simulink model "SHEST"  (R2022a)
settings: Solver=ode23tb  StartTime=0.0  StopTime=0.1  MaxStep=1e-3  RelTol=1e-2
undefined symbols (not defined in the file): DC_Source, Modulation_Index, phase_3_IGBTs, Sine_Wave, Three_Phase_RL
libraries: spsFourierLib x4, spsVoltageMeasurementLib x3, spsCurrentMeasurementLib x2, spsUniversalBridgeLib x1, spsDCVoltageSourceLib x1, spsMultimeterLib x1, spsPWMGenerator2LevelLib x1, spsRMSLib x1, spsThreePhaseSeriesRLCBranchLib x1, spspowerguiLib x1
settings Model: Creator=Student11  LastModifiedBy=админ
settings SolverCC: AlgebraicLoopSolver=TrustRegion
settings DataIOCC: ReturnWorkspaceOutputs=off
settings DebuggingCC: SFMachineParentedDataDiag=warning  ArithmeticOperatorsInVariantConditions=warning
settings SFSimCC: SimUseLocalCustomCode=off  CustomCodeUndefinedFunction=UseInterfaceOnly
settings RTWCC: RTWUseLocalCustomCode=off
settings CodeAppCC: StateflowObjectComments=on
settings SimscapeCC: SimscapeNormalizeSystem=off

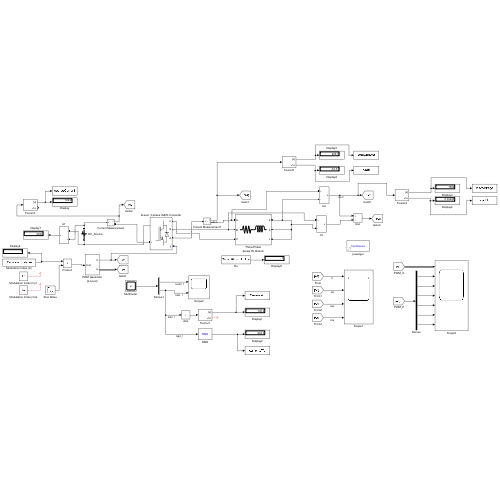
[thumbnail: Simulink's stored preview of the top-level diagram]
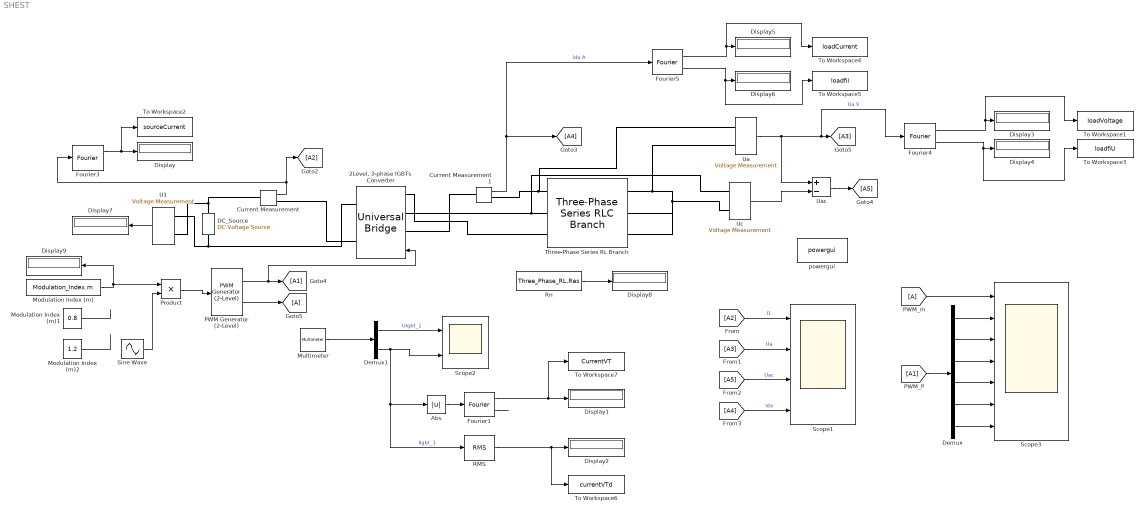
== system SHEST ==
  "2Level, 3-phase IGBTs Converter" : spsUniversalBridgeLib/Universal Bridge  Arms=3  SnubberResistance=phase_3_IGBTs.SnubberRs  SnubberCapacitance=phase_3_IGBTs.SnubberCs  Device=IGBT / Diodes  Ron=phase_3_IGBTs.R_on  Lon=0  ForwardVoltages=[phase_3_IGBTs.Vf phase_3_IGBTs.Vfd]  ForwardVoltage=[2 1]  GTOparameters=[ 10e-6 , 20e-6 ]  IGBTparameters=[ 1e-6 , 2e-6 ]  Measurements=All voltages and currents  Measurements_2=None  converterType=Rectifier
  Abs : Abs  SaturateOnIntegerOverflow=off
  Current Measurement : spsCurrentMeasurementLib/Current Measurement  PhasorSimulation=off  OutputType=Complex  PSBequivalent=0
  Current Measurement1 : spsCurrentMeasurementLib/Current Measurement  PhasorSimulation=off  OutputType=Complex  PSBequivalent=0
  DC_Source : spsDCVoltageSourceLib/DC Voltage Source  Amplitude=DC_Source.Voltage  Measurements=None
  Demux : Demux  Outputs=6
  Demux1 : Demux  Outputs=2
  Display{,1..9} (10 alike) : Display
  Fourier1 : spsFourierLib/Fourier  Freq=Fourier_1_4_5.frec  n=Fourier_1_4_5.harmonic  InInit=[0, 0]  Ts=0
      settings: SourceProductBaseCode=PS
  Fourier3 : spsFourierLib/Fourier  Freq=Fourier_3.frec  n=Fourier_3.harmonic  InInit=[0, 0]  Ts=0
      settings: SourceProductBaseCode=PS
  Fourier4 : spsFourierLib/Fourier  Freq=Fourier_1_4_5.frec  n=Fourier_1_4_5.harmonic  InInit=[0, 0]  Ts=0
      settings: SourceProductBaseCode=PS
  Fourier5 : spsFourierLib/Fourier  Freq=Fourier_1_4_5.frec  n=Fourier_1_4_5.harmonic  InInit=[0, 0]  Ts=0
      settings: SourceProductBaseCode=PS
  Goto5 : Goto
  Modulation Index (m) : Constant  Value=Modulation_Index.m
  Modulation Index (m)1 : Constant  Value=0.8
  Modulation Index (m)2 : Constant  Value=1.2
  Multimeter : spsMultimeterLib/Multimeter  L=16  sel=[1 11]  yselected={}  Gain=[1 1]  OutputType=Complex  PlotAtSimulationStop=off  PhasorSimulation=off
  PWM Generator (2-Level) : spsPWMGenerator2LevelLib/PWM Generator (2-Level)  ModulatorType=Three-phase bridge (6 pulses)  ModulatorMode=Unsynchronized  Fc=PWM_generator.frec  Pc=0  nF=27  MinMax="[ -1  1 ]"  SamplingTechnique=Natural  ModulatingSignals=off  m=0.8  Freq=60  Phase=0  Ts=0  ShowCarrierOutport=on
  PWM_m : From
  Product : Product
  RMS : spsRMSLib/RMS  TrueRMS=on  Freq=RMS_T.frec  RMSInit=0  Ts=0
  Rн : Constant  Value=Three_Phase_RL.Res
  Scope1 : Scope  NumInputPorts=4
  Scope2 : Scope  NumInputPorts=2
  Scope3 : Scope  NumInputPorts=7
  Sine Wave : Sin  Amplitude=Sine_Wave.amplitude  Frequency=Sine_Wave.freq  Phase=Sine_Wave.Phase  SampleTime=0
  Three-Phase Series RL Branch : spsThreePhaseSeriesRLCBranchLib/Three-Phase Series RLC Branch  LConnTagsString=A|B|C  RConnTagsString=A|B|C  BranchType=RL  Resistance=Three_Phase_RL.Res  Inductance=Three_Phase_RL.Ind  Capacitance=1e-6  Measurements=None
  To Workspace1 : ToWorkspace  VariableName=loadVoltage  SampleTime=-1
  To Workspace2 : ToWorkspace  VariableName=sourceCurrent  SampleTime=-1
  To Workspace3 : ToWorkspace  VariableName=loadfiU  SampleTime=-1
  To Workspace4 : ToWorkspace  VariableName=loadCurrent  SampleTime=-1
  To Workspace5 : ToWorkspace  VariableName=loadfiI  SampleTime=-1
  To Workspace6 : ToWorkspace  VariableName=currentVTd  SampleTime=-1
  To Workspace7 : ToWorkspace  VariableName=CurrentVT  SampleTime=-1
  U1 : spsVoltageMeasurementLib/Voltage Measurement  PhasorSimulation=off  OutputType=Complex  PSBequivalent=0
  Ua : spsVoltageMeasurementLib/Voltage Measurement  PhasorSimulation=off  OutputType=Complex  PSBequivalent=0
  Uac : Sum  Inputs=+-
  Uc : spsVoltageMeasurementLib/Voltage Measurement  PhasorSimulation=off  OutputType=Complex  PSBequivalent=0
  powergui : spspowerguiLib/powergui  Priority=1  SimulationMode=Continuous  SampleTime=50e-6  frequency=60  Iterations=50  frequencyindice=0  Pbase=100e6  ErrMax=1e-4  UnitsV=kV  UnitsW=MW  buscounter=0  FunctionMessages=off  echomessages=off  EnableUseOfTLC=off  CurrentSourceSwitches=off  DisableSnubberDevices=off  DisableRonSwitches=off  DisableVfSwitches=off  DisplayEquations=off  AutomaticDiscreteSolvers=off  SolverType=Tustin/Backward Euler (TBE)  Interpol=off  ExternalGateDelay=off  methode=off  Ts=100  x0status=blocks  SPID=on  SwTol=0  HookPort=off  NonlinearTolerance=1e-4  nMaxIteration=100  ContinueOnMaxIteration=off  RestoreLinks=warning  ResistiveCurrentMeasurement=off  Frange=[0:2:500]  Ylog=off  Xlog=on  ShowGrid=off  save=off  variable=ZData  structure=0  ZoomFFT=off  StartTime=0.0  cycles=1  DisplayStyle=1  fundamental=60  FreqAxis=off  MaxFrequency=1000  frequencyindicesteady=1  RmsSteady=1  display=off
  wires:
  [A5] -> Scope1/3  "Uac"
  [A3] -> Scope1/2  "Ua"
  [A2] -> Scope1/1  "I1"
  [A4] -> Scope1/4  "Ida"
  Current Measurement/1 -> Fourier3/1, [A2]
  Uc/1 -> Uac/2
  Ua/1 -> Uac/1, Fourier4/1, [A3]  "Ua V"
  Uac/1 -> [A5]
  Product/1 -> PWM Generator (2-Level)/1
  Sine Wave/1 -> Product/2
  PWM Generator (2-Level)/1 -> "2Level, 3-phase IGBTs Converter"/1, [A1]
  PWM Generator (2-Level)/2 -> Goto5/1
  Fourier3/1 -> To Workspace2/1, Display/1
  PWM_m/1 -> Scope3/1
  [A1] -> Demux/1
  Demux/1 -> Scope3/2
  Demux/2 -> Scope3/3
  Demux/3 -> Scope3/4
  Demux/4 -> Scope3/5
  Demux/5 -> Scope3/6
  Demux/6 -> Scope3/7
  Multimeter/1 -> Demux1/1
  Demux1/1 -> Scope2/1  "Uigbt_1"
  Demux1/2 -> Abs/1, RMS/1, Scope2/2  "Iigbt_1"
  RMS/1 -> To Workspace6/1, Display2/1
  Fourier1/1 -> To Workspace7/1, Display1/1
  Abs/1 -> Fourier1/1
  Fourier4/1 -> To Workspace1/1, Display3/1
  Fourier4/2 -> To Workspace3/1, Display4/1
  Fourier5/1 -> Display5/1, To Workspace4/1
  Fourier5/2 -> To Workspace5/1, Display6/1
  Rн/1 -> Display8/1
  Current Measurement1/1 -> [A4], Fourier5/1  "ida A"
  U1/1 -> Display7/1
  Fourier1/2 -> ?
  Modulation Index (m)/1 -> Product/1, Display9/1
  Modulation Index (m)1/1 -> ?
  Modulation Index (m)2/1 -> ?
  connections:
  DC_Source/RConn1 -- U1/LConn1 -- Current Measurement/LConn1
  DC_Source/LConn1 -- "2Level, 3-phase IGBTs Converter"/RConn2 -- U1/LConn2
  "2Level, 3-phase IGBTs Converter"/LConn2 -- Uc/LConn1 -- Three-Phase Series RL Branch/LConn2
  "2Level, 3-phase IGBTs Converter"/LConn3 -- Three-Phase Series RL Branch/LConn3
  "2Level, 3-phase IGBTs Converter"/LConn1 -- Current Measurement1/LConn1
  Current Measurement1/RConn1 -- Ua/LConn1 -- Three-Phase Series RL Branch/LConn1
  Three-Phase Series RL Branch/RConn1 -- Three-Phase Series RL Branch/RConn3 -- Three-Phase Series RL Branch/RConn2 -- Uc/LConn2 -- Ua/LConn2
  "2Level, 3-phase IGBTs Converter"/RConn1 -- Current Measurement/RConn1
